simulink model "SSR_IFFT"  (R2023b)
settings: Solver=VariableStepAuto  StartTime=0.0  StopTime=2E-9*N/SSR*8  RelTol=1e-3
PreLoadFcn:
  | N=1024;
  | SSR=4;
undefined symbols (not defined in the file or in its folder): Low
libraries: hdlBasic x9, hdlSSR x5, dspbuff3 x1, hdlUtilities x1, dspxfrm3 x1, dspswit3 x1, vmcUtilities x1
settings Model: Creator=admin  LastModifiedBy=Jakub
settings SolverCC: AlgebraicLoopSolver=TrustRegion
settings DataIOCC: ReturnWorkspaceOutputs=off
settings DebuggingCC: UnconnectedInputMsg=warning  UnconnectedOutputMsg=warning  UnconnectedLineMsg=warning  ArithmeticOperatorsInVariantConditions=warning
settings ModelReferenceCC: EnableRefExpFcnMdlSchedulingChecks=on
settings SFSimCC: SimUseLocalCustomCode=off  CustomCodeUndefinedFunction=UseInterfaceOnly
settings RTWCC: RTWUseLocalCustomCode=off  DLArmComputeVersion=19.05
settings CodeAppCC: StateflowObjectComments=on

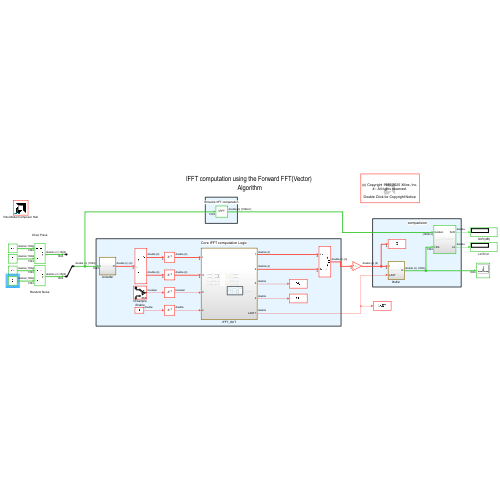
[thumbnail: Simulink's stored preview of the top-level diagram]
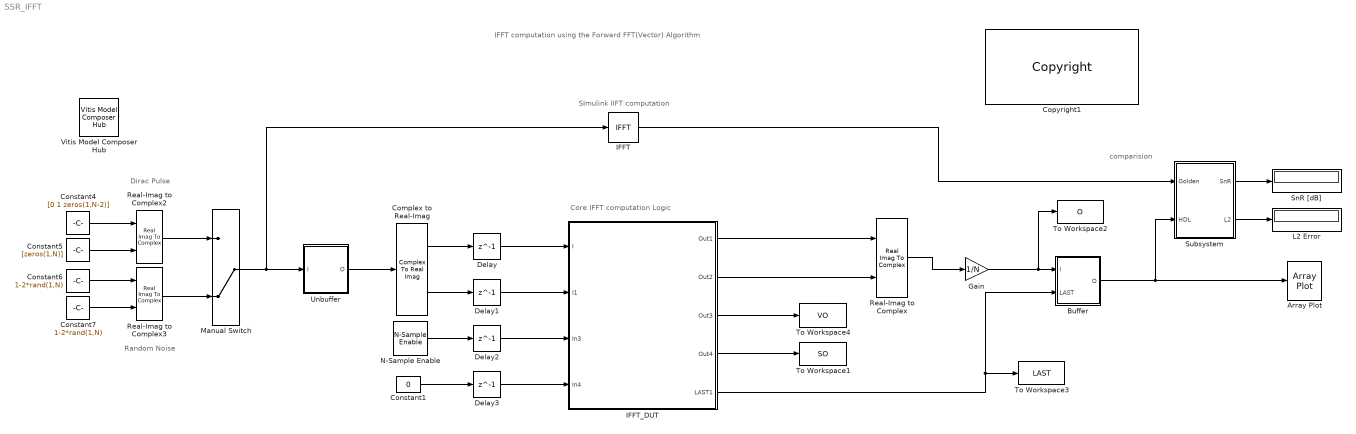
== system SSR_IFFT ==
  note: comparision
  note: SImulink IIFT computation
  note: Core IFFT computation Logic
  note: Dirac Pulse
  note: Random Noise
  note: IFFT computation using the Forward FFT(Vector)
      | Algorithm
  Array Plot : ArrayPlot  WindowPosition=[1068.000000,318.000000,724.000000,431.000000,]  ShowLegend=on  DefaultConfigurationName=dsp.scopes.ArrayPlotBlockSpecification
  Buffer : Subsystem
  Complex to Real-Imag : ComplexToRealImag
  Constant1 : Constant  Value=0  SampleTime=-1
  Constant4 : Constant  Value=[0 1 zeros(1,N-2)]  SampleTime=-1
  Constant5 : Constant  Value=[zeros(1,N)]  SampleTime=-1
  Constant6 : Constant  Value=1-2*rand(1,N)  SampleTime=-1
  Constant7 : Constant  Value=1-2*rand(1,N)  SampleTime=-1
  Copyright1 : hdlUtilities/Copyright  copyrighttext="Copyright (c) 2025  by  Xilinx, Inc. All rights reserved.<br><br>This file contains proprietary, confidential information of Xilinx, Inc., is distributed under license from Xilinx, Inc., and may be used, copied and/or disclosed only pursuant to the terms of a valid license agreement with Xilinx, Inc. Xilinx hereby grants you a license to use this file solely for design, simulation, implementation and creation of design files limited to Xilinx devices or technologies. Use with non-Xilinx devices or technologies is expressly prohibited and immediately terminates your license unless covered by a separate agreement.<br><br>Xilinx is providing this design, code, or information \"as-is\" solely for use in developing programs and solutions for Xilinx devices, with no obligation on the part of Xilinx to provide support. By providing this design, code, or information as one possible implementation of this feature, application or standard, Xilinx is making no representation that this implementation is free from any claims of infringement. You are responsible for obtaining any rights you may require for your implementation. Xilinx expressly disclaims any warranty whatsoever with respect to the adequacy of the implementation, including but not limited to any warranties or representations that this implementation is free from claims of infringement, implied warranties of merchantability or fitness for a particular purpose.<br><br>Xilinx products are not intended for use in life support appliances, devices, or systems. Use in such applications is expressly prohibited.<br><br>Any modifications that are made to the Source Code are done at the user's sole risk and will be unsupported.<br><br>This copyright and support notice must be retained as part of this text at all times. (c) Copyright 1995-2025 Xilinx, Inc. All rights reserved."  block_type=copyright
  Delay{,1..3} (4 alike) : Delay  DelayLength=1
  Gain : Gain  Gain=1/N
  IFFT : dspxfrm3/IFFT  FFTImplementation=FFTW  CompMethod=Table lookup  TableOpt=NEW  TableOptActive=Speed  BitRevOrder=off  cs_in=off  Normalize=on  InheritFFTLength=on  FFTLength=64  WrapInput=on  mode=Complex  outSamplingMode=Sample based  roundingMode=Floor  overflowMode=off  firstCoeffDataTypeStr=Inherit: Same word length as input  firstCoeffLastDataTypeStr=Inherit: Same word length as input  outputMin=[]  outputMax=[]
  IFFT_DUT : Subsystem
  L2 Error : Display
  Manual Switch : ManualSwitch  CurrentSetting=0
  N-Sample Enable : dspswit3/N-Sample Enable  N=N/SSR  ActiveLevel=Low (0)  reset=off  TriggerType=Rising edge  Ts=-1  DataType=Logical
  Real-Imag to Complex : RealImagToComplex
  Real-Imag to Complex2 : RealImagToComplex
  Real-Imag to Complex3 : RealImagToComplex
  SnR [dB] : Display
  Subsystem : Subsystem
  To Workspace1 : ToWorkspace  VariableName=SO  SampleTime=-1
  To Workspace2 : ToWorkspace  VariableName=O  SampleTime=-1
  To Workspace3 : ToWorkspace  VariableName=LAST  SampleTime=-1
  To Workspace4 : ToWorkspace  VariableName=VO  SampleTime=-1
  Unbuffer : Subsystem
  Vitis Model Composer Hub : vmcUtilities/Vitis Model Composer Hub  Tag=genX  CodeGeneration=off  SubsystemName=IFFT_DUT  TargetDirectory=./code  exportDesign=off  analyzeDesign=off  validateDesignOnHw=off  ExportType=System Generator  IpVendor=xilinx.com  IpLibrary=hls  IpVersion=1.0  IpHWLanguage=Verilog  AieCompilerOptions={}  AieSimulatorOptions={}  CreateTestbench=off  TestbenchStackSize=10  RunRtlSim=off  RunCSim=off  RunAieSim=off  AieSimTimeout=50000  RunAieSimProfiling=off  LaunchVitisAnalyzer=off  PlotOutput=off  RunX86Sim=off  X86SimTimeout=10  GenHwImage=off  GenLibadfXo=on  GenHwValidationCode=off  PlatformType=Not Specified  HwSystemType=Baremetal  HwValidationTarget=hw  ProjDevice=Zynq UltraScale+ ZCU111 Evaluation Platform (xczu28dr-ffvg1517-2-e)  ProjDevicePart=xczu28dr-ffvg1517-2-e  AIEType=None  SamplePeriod=-1  ClockFrequency=200  DataPathParallelism=1  xilinxfamily=zynquplusRFSOC  part=xczu28dr  speed=-2-e  package=ffvg1517  directory=./netlist\ip\IFFT_DUT\src  testbench=off  incr_netlist=off  synthesis_tool=Vivado  clock_wrapper=Clock Enables  dbl_ovrd=According to Block Masks  dcm_input_clock_period=10  sysclk_period=2  simulink_period=2E-09  eval_field=0  IPInfoJsonString="{\"HDLSubsystem\":{\"SubsystemName\":\"IFFT_DUT\",\"IPName\":\"IFFT_DUT\",\"IPLibrary\":\"VMC\",\"IPVendor\":\"User Company\",\"IPVersion\":\"1.0\"}}"  LogFileName=''  NThreads=4
  wires:
  Constant1/1 -> Delay3/1
  Complex to Real-Imag/2 -> Delay1/1
  N-Sample Enable/1 -> Delay2/1
  Real-Imag to Complex2/1 -> Manual Switch/1
  Constant4/1 -> Real-Imag to Complex2/1
  Constant5/1 -> Real-Imag to Complex2/2
  Constant7/1 -> Real-Imag to Complex3/2
  Constant6/1 -> Real-Imag to Complex3/1
  Real-Imag to Complex3/1 -> Manual Switch/2
  Manual Switch/1 -> IFFT/1, Unbuffer/1(I)
  Buffer/1(O) -> Array Plot/1, Subsystem/2(HDL)
  Real-Imag to Complex/1 -> Gain/1
  Subsystem/1(SnR) -> SnR [dB]/1
  Subsystem/2(L2) -> L2 Error/1
  Complex to Real-Imag/1 -> Delay/1
  Unbuffer/1(O) -> Complex to Real-Imag/1
  IFFT/1 -> Subsystem/1(Golden)
  Gain/1 -> To Workspace2/1, Buffer/1(I)
  Delay/1 -> IFFT_DUT/1(I)
  Delay1/1 -> IFFT_DUT/2(I1)
  Delay2/1 -> IFFT_DUT/3(In3)
  Delay3/1 -> IFFT_DUT/4(In4)
  IFFT_DUT/1(Out1) -> Real-Imag to Complex/1
  IFFT_DUT/2(Out2) -> Real-Imag to Complex/2
  IFFT_DUT/3(Out3) -> To Workspace4/1
  IFFT_DUT/4(Out4) -> To Workspace1/1
  IFFT_DUT/5(LAST1) -> Buffer/2(LAST), To Workspace3/1

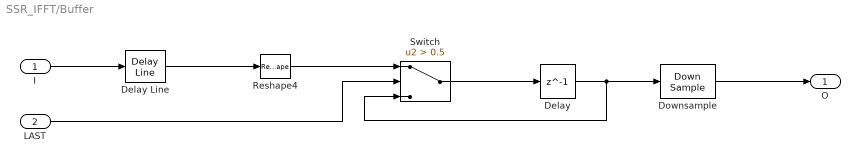
== system SSR_IFFT/Buffer ==
  I : Inport
  LAST : Inport  Port=2
  Delay : Delay  DelayLength=1
  Delay Line : dspbuff3/Delay Line  siz=N  ic=0  directfeed=off  enable_output=off  hold_output=off  OutputFrames=off
  Downsample : DownSample  N=N/SSR  RateOptions=Allow multirate processing
  Reshape4 : Reshape  OutputDimensions=[256,4]
  Switch : Switch  Criteria=u2 > Threshold  Threshold=0.5  SaturateOnIntegerOverflow=off  InputSameDT=off
  O : Outport  VectorParamsAs1DForOutWhenUnconnected=off
  wires:
  Switch/1 -> Delay/1
  I/1 -> Delay Line/1
  Downsample/1 -> O/1
  Delay/1 -> Switch/3, Downsample/1
  Delay Line/1 -> Reshape4/1
  Reshape4/1 -> Switch/1
  LAST/1 -> Switch/2

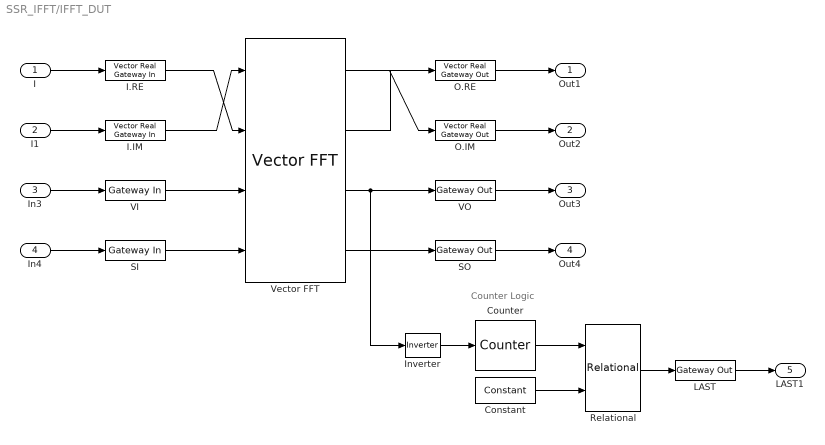
== system SSR_IFFT/IFFT_DUT ==
  note: Counter Logic
  I : Inport
  I1 : Inport  Port=2
  In3 : Inport  Port=3
  In4 : Inport  Port=4
  Constant : hdlBasic/Constant  const=N/SSR-1  gui_display_data_type=Fixed-point  arith_type=Unsigned  n_bits=log2(N/SSR)  bin_pt=0  preci_type=Single  exp_width=8  frac_width=24  explicit_period=off  period=1  XmcBlockStatus=1  maskContainerNames=tabcontainer1  block_type=constant  block_config=sysgen:Constant_config
  Counter : hdlBasic/Counter  cnt_type=Free running  cnt_to=Inf  operation=Up  start_count=0  cnt_by_val=1  arith_type=Unsigned  n_bits=log2(N/SSR)  bin_pt=0  load_pin=off  rst=on  en=off  explicit_period=Explicit  period=2E-9  use_behavioral_HDL=off  implementation=Fabric  XmcBlockStatus=1  maskContainerNames=group1  block_type=counter  block_config=sysgen:Counter_config  block_width=531  block_height=1023
  I.IM : hdlSSR/Vector Real Gateway In  gui_display_data_type=Fixed-point  arith_type=Signed (2's comp)  n_bits=18  bin_pt=16  preci_type=Single  exp_width=8  frac_width=24  quantization="Round  (unbiased: +/- Inf)"  overflow=Saturate  period=2E-9  sg_ssr=SSR  UseAsADC=off  ADCChannel='1'  interface=None  automatic_assignment=off  address_offset=hex2dec('00')  intf_name=''  intf_description=''  default_value=0  timing_constraint=None  locs_specified=off  LOCs={}  io_standard={}  inherit_from_input=off  hdl_port=on  interface_prev=1  block_type=realgatewayin_ssr  XmcBlockStatus=1  sg_ssr_prev=4  maskContainerNames=group4  block_width_w=590  block_height_w=670  block_width=640  block_height=850
  I.RE : hdlSSR/Vector Real Gateway In  gui_display_data_type=Fixed-point  arith_type=Signed (2's comp)  n_bits=18  bin_pt=16  preci_type=Single  exp_width=8  frac_width=24  quantization="Round  (unbiased: +/- Inf)"  overflow=Saturate  period=2E-9  sg_ssr=SSR  UseAsADC=off  ADCChannel='1'  interface=None  automatic_assignment=off  address_offset=hex2dec('00')  intf_name=''  intf_description=''  default_value=0  timing_constraint=None  locs_specified=off  LOCs={}  io_standard={}  inherit_from_input=off  hdl_port=on  interface_prev=1  block_type=realgatewayin_ssr  XmcBlockStatus=1  sg_ssr_prev=4  maskContainerNames=group4  block_width_w=590  block_height_w=670  block_width=640  block_height=850
  Inverter : hdlBasic/Inverter  en=off  latency=0  XmcBlockStatus=1  maskContainerNames=group2  block_type=inv  block_config=sysgen:Inverter_config
  LAST : hdlBasic/Gateway Out  inherit_from_input=off  hdl_port=on  rows=1  columns=1  UseAsDAC=off  DACChannel='1'  interface=None  automatic_assignment=on  address_offset=hex2dec('00')  intf_name=''  intf_description=''  timing_constraint=None  locs_specified=off  LOCs={}  io_standard={}  XmcBlockStatus=1  maskContainerNames=group4  block_type=gatewayout  block_config=sysgen:gateway_out_config  block_width_w=590  block_height_w=620  block_width=620  block_height=750
  O.IM : hdlSSR/Vector Real Gateway Out  inherit_from_input=off  hdl_port=on  sg_ssr=SSR  rows=1  columns=1  UseAsDAC=off  DACChannel='1'  interface=None  automatic_assignment=on  address_offset=hex2dec('00')  intf_name=''  intf_description=''  timing_constraint=None  locs_specified=off  LOCs={}  io_standard={}  block_type=realgatewayout_ssr  XmcBlockStatus=1  sg_ssr_prev=4  maskContainerNames=group4  block_width_w=590  block_height_w=620  block_width=620  block_height=750
  O.RE : hdlSSR/Vector Real Gateway Out  inherit_from_input=off  hdl_port=on  sg_ssr=SSR  rows=1  columns=1  UseAsDAC=off  DACChannel='1'  interface=None  automatic_assignment=on  address_offset=hex2dec('00')  intf_name=''  intf_description=''  timing_constraint=None  locs_specified=off  LOCs={}  io_standard={}  block_type=realgatewayout_ssr  XmcBlockStatus=1  sg_ssr_prev=4  maskContainerNames=group4  block_width_w=590  block_height_w=620  block_width=620  block_height=750
  Relational : hdlBasic/Relational  mode=a=b  op_type=Bool  en=off  latency=1  XmcBlockStatus=1  maskContainerNames=tabcontainer1  block_type=relational  block_config=sysgen:Relational_config
  SI : hdlBasic/Gateway In  gui_display_data_type=Fixed-point  arith_type=Unsigned  n_bits=log2(N)  bin_pt=0  preci_type=Single  exp_width=8  frac_width=24  rows=1  columns=1  quantization="Round  (unbiased: +/- Inf)"  overflow=Saturate  period=2E-9  UseAsADC=off  ADCChannel='1'  interface=None  automatic_assignment=on  address_offset=hex2dec('00')  intf_name=''  intf_description=''  default_value=0  timing_constraint=None  locs_specified=off  LOCs={}  io_standard={}  inherit_from_input=off  hdl_port=on  XmcBlockStatus=1  maskContainerNames=group4  block_type=gatewayin  block_config=sysgen:gateway_in_config  block_width_w=590  block_height_w=620  block_width=640  block_height=850
  SO : hdlBasic/Gateway Out  inherit_from_input=off  hdl_port=on  rows=1  columns=1  UseAsDAC=off  DACChannel='1'  interface=None  automatic_assignment=on  address_offset=hex2dec('00')  intf_name=''  intf_description=''  timing_constraint=None  locs_specified=off  LOCs={}  io_standard={}  XmcBlockStatus=1  maskContainerNames=group4  block_type=gatewayout  block_config=sysgen:gateway_out_config  block_width_w=590  block_height_w=620  block_width=620  block_height=750
  VI : hdlBasic/Gateway In  gui_display_data_type=Boolean  arith_type=Boolean  n_bits=16  bin_pt=14  preci_type=Single  exp_width=8  frac_width=24  rows=1  columns=1  quantization="Round  (unbiased: +/- Inf)"  overflow=Saturate  period=2E-9  UseAsADC=off  ADCChannel='1'  interface=None  automatic_assignment=on  address_offset=hex2dec('00')  intf_name=''  intf_description=''  default_value=0  timing_constraint=None  locs_specified=off  LOCs={}  io_standard={}  inherit_from_input=off  hdl_port=on  XmcBlockStatus=1  maskContainerNames=group4  block_type=gatewayin  block_config=sysgen:gateway_in_config  block_width_w=590  block_height_w=620  block_width=640  block_height=850
  VO : hdlBasic/Gateway Out  inherit_from_input=off  hdl_port=on  rows=1  columns=1  UseAsDAC=off  DACChannel='1'  interface=None  automatic_assignment=on  address_offset=hex2dec('00')  intf_name=''  intf_description=''  timing_constraint=None  locs_specified=off  LOCs={}  io_standard={}  XmcBlockStatus=1  maskContainerNames=group4  block_type=gatewayout  block_config=sysgen:gateway_out_config  block_width_w=590  block_height_w=620  block_width=620  block_height=750
  Vector FFT : hdlSSR/Vector FFT  N=N  n_bits=26  bin_pt=16  rounding=on  bypass_input_swap=off  bypass_ouput_dsn=off  bram_threshold=258  use_cm4=3  use_cb=off  sg_ssr=SSR  block_type=fft_ssr  W_high=1  W_low=-17  XmcBlockStatus=1  sg_ssr_prev=4  maskContainerNames=group3
  Out1 : Outport
  Out2 : Outport  Port=2
  Out3 : Outport  Port=3
  Out4 : Outport  Port=4
  LAST1 : Outport  Port=5
  wires:
  I/1 -> I.RE/1
  I1/1 -> I.IM/1
  VO/1 -> Out3/1
  I.IM/1 -> Vector FFT/1
  I.RE/1 -> Vector FFT/2
  In3/1 -> VI/1
  SO/1 -> Out4/1
  O.RE/1 -> Out1/1
  Vector FFT/2 -> O.RE/1
  In4/1 -> SI/1
  VI/1 -> Vector FFT/3
  O.IM/1 -> Out2/1
  SI/1 -> Vector FFT/4
  Vector FFT/1 -> O.IM/1
  Vector FFT/4 -> SO/1
  Constant/1 -> Relational/2
  Counter/1 -> Relational/1
  Vector FFT/3 -> Inverter/1, VO/1
  Relational/1 -> LAST/1
  Inverter/1 -> Counter/1
  LAST/1 -> LAST1/1

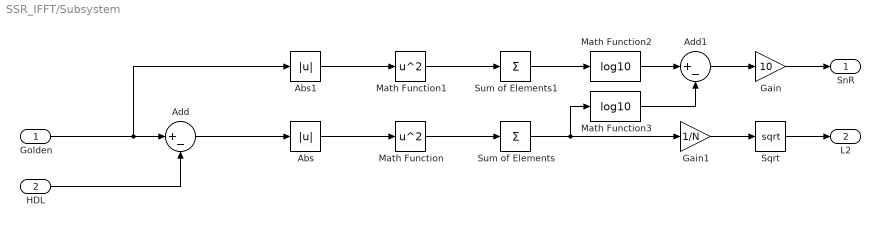
== system SSR_IFFT/Subsystem ==
  Golden : Inport
  HDL : Inport  Port=2
  Abs : Abs  SaturateOnIntegerOverflow=off
  Abs1 : Abs  SaturateOnIntegerOverflow=off
  Add : Sum  Inputs=|+-
  Add1 : Sum  Inputs=|+-
  Gain : Gain  Gain=10
  Gain1 : Gain  Gain=1/N
  Math Function : Math  Operator=square  SignedPower=on
  Math Function1 : Math  Operator=square  SignedPower=on
  Math Function2 : Math  Operator=log10  SignedPower=on
  Math Function3 : Math  Operator=log10  SignedPower=on
  Sqrt : Sqrt
  Sum of Elements : Sum  Inputs=+
  Sum of Elements1 : Sum  Inputs=+
  SnR : Outport  VectorParamsAs1DForOutWhenUnconnected=off
  L2 : Outport  Port=2  VectorParamsAs1DForOutWhenUnconnected=off
  wires:
  Gain/1 -> SnR/1
  Add1/1 -> Gain/1
  Math Function3/1 -> Add1/2
  Math Function1/1 -> Sum of Elements1/1
  Sum of Elements1/1 -> Math Function2/1
  Abs1/1 -> Math Function1/1
  Math Function/1 -> Sum of Elements/1
  Sum of Elements/1 -> Math Function3/1, Gain1/1
  Golden/1 -> Abs1/1, Add/1
  Math Function2/1 -> Add1/1
  Abs/1 -> Math Function/1
  Add/1 -> Abs/1
  HDL/1 -> Add/2
  Sqrt/1 -> L2/1
  Gain1/1 -> Sqrt/1

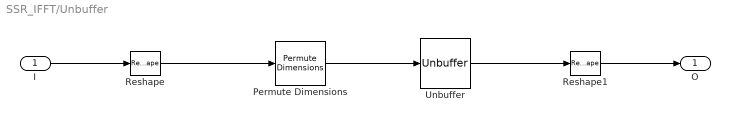
== system SSR_IFFT/Unbuffer ==
  I : Inport
  Permute Dimensions : PermuteDimensions
  Reshape : Reshape  OutputDimensionality=Customize  OutputDimensions=[SSR,N/SSR]
  Reshape1 : Reshape  OutputDimensions=[256,4]
  Unbuffer : Unbuffer
  O : Outport  VectorParamsAs1DForOutWhenUnconnected=off
  wires:
  Unbuffer/1 -> Reshape1/1
  Permute Dimensions/1 -> Unbuffer/1
  Reshape/1 -> Permute Dimensions/1
  Reshape1/1 -> O/1
  I/1 -> Reshape/1
